simulink subsystem "Enviar_Dados_para_MCU"  (R2023b)
settings: Solver=VariableStepAuto  StartTime=0.0  StopTime=10.0  RelTol=1e-3
settings Model: Creator=Ricardo  LastModifiedBy=Ricardo

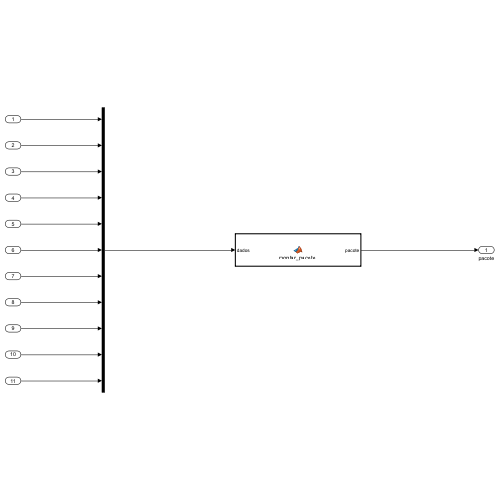
[thumbnail: Simulink's stored preview of the top-level diagram]
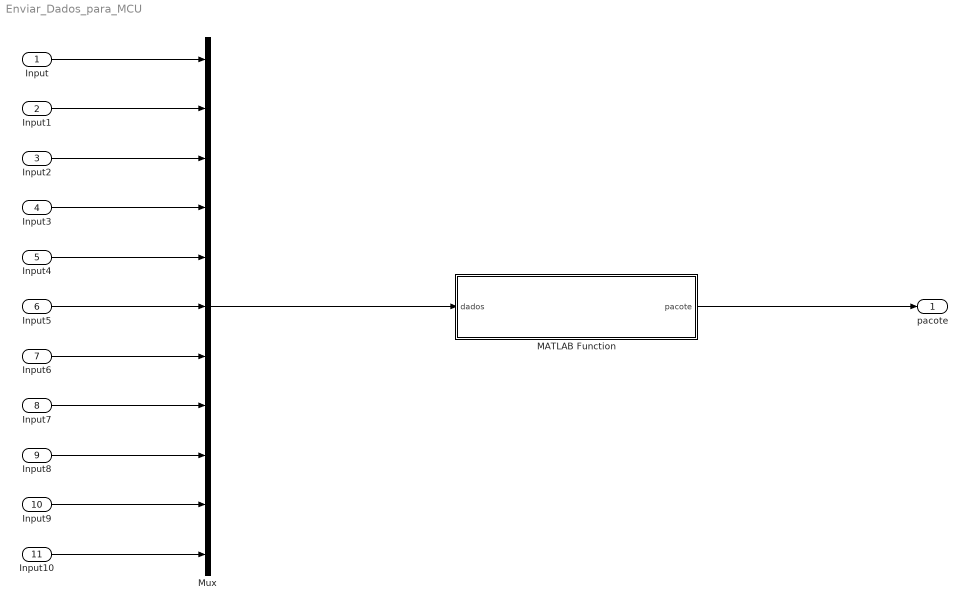
== system Enviar_Dados_para_MCU ==
  Input : Inport
  Input1 : Inport  Port=2
  Input2 : Inport  Port=3
  Input3 : Inport  Port=4
  Input4 : Inport  Port=5
  Input5 : Inport  Port=6
  Input6 : Inport  Port=7
  Input7 : Inport  Port=8
  Input8 : Inport  Port=9
  Input9 : Inport  Port=10
  Input10 : Inport  Port=11
  MATLAB Function : MATLAB Function  TreatAsAtomicUnit=on
  Mux : Mux  Inputs=11
  pacote : Outport
  wires:
  Input/1 -> Mux/1
  Input1/1 -> Mux/2
  Input2/1 -> Mux/3
  Input3/1 -> Mux/4
  Input4/1 -> Mux/5
  Input5/1 -> Mux/6
  Input6/1 -> Mux/7
  Input7/1 -> Mux/8
  Input8/1 -> Mux/9
  Input9/1 -> Mux/10
  Input10/1 -> Mux/11
  Mux/1 -> MATLAB Function/1(dados)
  MATLAB Function/1(pacote) -> pacote/1

== matlab function Enviar_Dados_para_MCU/MATLAB Function ==
  data: dados input; pacote output
function pacote = montar_pacote(dados)
    START_BYTE = uint8(170); % 0xAA
    PACKET_TYPE = uint8(1);  % 0x01 para entrada
    END_BYTE = uint8(85);    % 0x55

    % Garante que dados seja um vetor coluna de 11 elementos
    dados = reshape(dados, [], 1);
    if length(dados) ~= 11
        error('Número incorreto de entradas. Esperado: 11');
    end

    % Converte dados para bytes
    dados_bytes = typecast(dados, 'uint8');
    comprimento = uint8(length(dados_bytes));

    % Verifica se o comprimento dos dados_bytes é 88 (11*8)
    if comprimento ~= 88
        error('Comprimento dos dados bytes incorreto. Esperado: 88');
    end

    % Pré-aloca o pacote com o tamanho correto (93 bytes)
    pacote = zeros(93, 1, 'uint8');

    % Monta o pacote
    pacote(1) = START_BYTE;
    pacote(2) = PACKET_TYPE;
    pacote(3) = comprimento;
    pacote(4:4+length(dados_bytes)-1) = dados_bytes;

    % Calcula e adiciona o checksum
    checksum = uint8(mod(sum(pacote(2:end-2)), 256));
    pacote(end-1) = checksum;
    pacote(end) = END_BYTE;
end
